simulink model "DA62_control"  (R2021a)
settings: Solver=ode4  StartTime=0.0  StopTime=300  FixedStep=0.001  RelTol=1e-3
InitFcn:
  | run('Stability_DA62')
values from neighbouring files (symbols this model uses):
  A = [Xu Xw 0 -g; Zu Zw U1 0; Mu+Mwdot*Zu Mw+Mwdot*Zw Mq+Mwdot*U1 0; 0 0 1 0]    [Stability_DA62.m]
  A_Lateral = [ Y_beta/U1 Y_p/U1 -(1-(Y_r/U1)) g*cosd(2)/U1 0; L_beta L_p L_r 0 0; N_beta N_p N_r 0 0; 0 1 0 0 0;0 0 1 0 0]    [Stability_DA62.m]
  B = [XdeltaE ;ZdeltaE; MdeltaE+Mwdot*ZdeltaE; 0]    [Stability_DA62.m]
  B_lateral = [Ydelta_a/U1 Ydelta_r/U1;Ldelta_a Ldelta_r; Ndelta_a Ndelta_r; 0 0;0 0 ]    [Stability_DA62.m]
  C_lateral = eye(5)    [Stability_DA62.m]
undefined symbols (not defined in the file or in its folder): Klqrgains
libraries: pid_lib x1
settings Model: Creator=IT-Defenders  LastModifiedBy=IT-Defenders

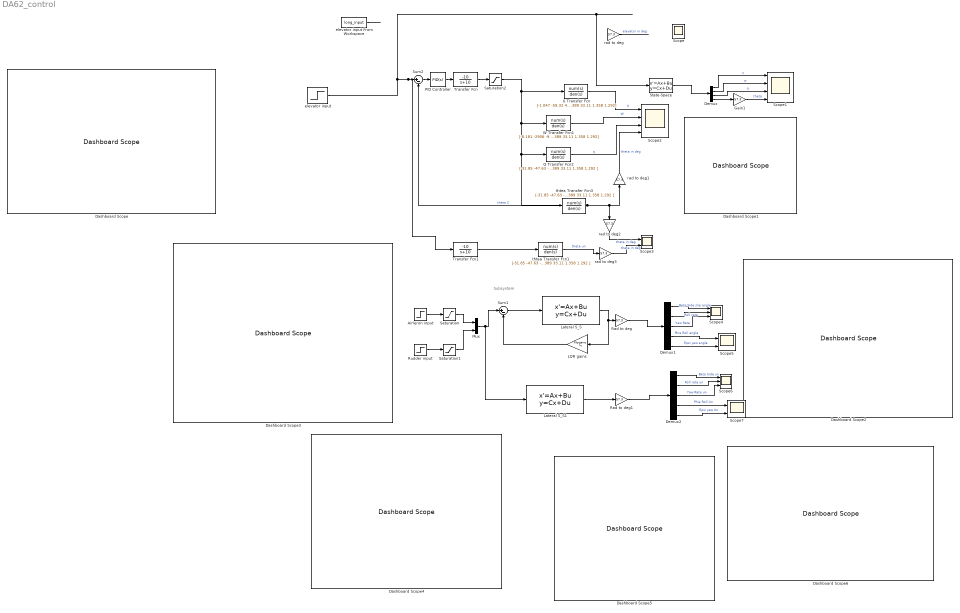
== system DA62_control ==
  note: Subsystem
  Airleron input : Step  After=20*pi/180  SampleTime=0
  Dashboard Scope{,1..6} (7 alike) : DashboardScope
  Demux : Demux
  Demux1 : Demux  Outputs=5
  Demux2 : Demux  Outputs=5
  Gain1 : Gain  Gain=57.3
  LQR gains : Gain  Gain=Klqrgains  Multiplication=Matrix(K*u)
  Lateral S_S : StateSpace  A=A_Lateral  B=B_lateral  C=C_lateral  D=zeros(5,2)  InitialCondition=0
  Lateral S_S1 : StateSpace  A=A_Lateral  B=B_lateral  C=C_lateral  D=zeros(5,2)  InitialCondition=0
  Mux : Mux  Inputs=2
  PID Controller : pid_lib/PID Controller  Controller=PID  Form=Parallel  TimeDomain=Continuous-time  UseExternalTs=off  SampleTime=-1  IntegratorMethod=Forward Euler  FilterMethod=Forward Euler  ControllerParametersSource=internal  P=0.880006891357761  I=0.782288298555866  D=-0.00238096460358231  UseFilter=on  N=369.600997021852  TunerSelectOption=Transfer Function Based (PID Tuner App)  InitialConditionSource=internal  InitialConditionForIntegrator=0  InitialConditionForFilter=0  DifferentiatorICPrevScaledInput=0  ExternalReset=none  TrackingMode=off  Kt=1  LimitOutput=off  SatLimitsSource=internal  UpperSaturationLimit=inf  LowerSaturationLimit=-inf  LinearizeAsGain=on  AntiWindupMode=none  Kb=1  POutMin=[]  POutMax=[]  IOutMin=[]  IOutMax=[]  DOutMin=[]  DOutMax=[]  NOutMin=[]  NOutMax=[]  SumOutMin=[]  SumOutMax=[]  SaturationOutMin=[]  SaturationOutMax=[]  PParamMin=[]  PParamMax=[]  IParamMin=[]  IParamMax=[]  DParamMin=[]  DParamMax=[]  NParamMin=[]  NParamMax=[]  KbParamMin=[]  KbParamMax=[]  KtParamMin=[]  KtParamMax=[]  KbOutMin=[]  KbOutMax=[]  KtOutMin=[]  KtOutMax=[]  IntegratorOutMin=[]  IntegratorOutMax=[]  FilterOutMin=[]  FilterOutMax=[]  SumI1OutMin=[]  SumI1OutMax=[]  SumI2OutMin=[]  SumI2OutMax=[]  SumI3OutMin=[]  SumI3OutMax=[]  SumI4OutMin=[]  SumI4OutMax=[]  SumDOutMin=[]  SumDOutMax=[]  DifferentiatorOutMin=[]  DifferentiatorOutMax=[]  FilterDiffOutCoefMin=[]  FilterDiffOutCoefMax=[]  ReciprocalOutMin=[]  ReciprocalOutMax=[]  SumDenOutMin=[]  SumDenOutMax=[]  SumNumOutMin=[]  SumNumOutMax=[]  DivideOutMin=[]  DivideOutMax=[]  UdiffTsProdOutMin=[]  UdiffTsProdOutMax=[]  NTsProdOutMin=[]  NTsProdOutMax=[]  UintegralTsProdOutMin=[]  UintegralTsProdOutMax=[]  UngainTsProdOutMin=[]  UngainTsProdOutMax=[]  IntegratorContinuousStateAttributes=''  IntegratorStateMustResolveToSignalObject=off  IntegratorRTWStateStorageClass=Auto  FilterContinuousStateAttributes=''  FilterStateMustResolveToSignalObject=off  FilterRTWStateStorageClass=Auto  ParallelPVariant=InternalParameters  IdealPVariant=Disabled  IVariant=InternalParameters  DVariant=InternalParameters  IntegratorVariant=Continuous  SatVariant=Disabled  AWVariant=Passthrough  PCopyVariant=Disabled  TRVariant=Disabled  FdbkBlocksVariant=Forward  IdealPFdbkVariant=Disabled  SatFdbkVariant=Disabled  DerivativeFilterVariant=ContFilter  NVariant=InternalParameters  NCopyVariant=Disabled  FilterICVariant=InternalICsFilter  IntegratorICVariant=InternalICs  ExternalResetVariant=Disabled  TRSumVariant=Passthrough  SumFdbkVariant=Disabled  SumVariant=Sum_PID  TsampFilterVariant=InternalTs  TsampNgainVariant=Passthrough  TsampIntegralVariant=Passthrough  ExternalSaturationOutDataTypeStr=Inherit: Same as second input
  Q Transfer Fcn2 : TransferFcn  Numerator=[-31.85 -47.63 -3.34 0]  Denominator=[1 6.389 33.11 1.358 1.292 ]
  Rad to deg : Gain  Gain=57.3
  Rad to deg1 : Gain  Gain=57.3
  Rudder input : Step  After=30*pi/180  SampleTime=0
  Saturation : Saturate  UpperLimit=50*pi/180  LowerLimit=-50*pi/180
  Saturation1 : Saturate  UpperLimit=30*pi/180  LowerLimit=-30*pi/180
  Saturation2 : Saturate  UpperLimit=15*pi/180  LowerLimit=-18*pi/180
  Scope{,3,5,7} (4 alike) : Scope  NumInputPorts=2
  Scope1 : Scope  NumInputPorts=4
  Scope2 : Scope  NumInputPorts=4
  Scope4 : Scope  NumInputPorts=3
  Scope6 : Scope  NumInputPorts=3
  State-Space : StateSpace  A=A  B=B  C=eye(4)  D=[0;0;0;0]  InitialCondition=0
  Sum1 : Sum  Inputs=|+-
  Sum2 : Sum  Inputs=|+-
  Transfer Fcn : TransferFcn  Numerator=[-10]  Denominator=[1 10]
  Transfer Fcn1 : TransferFcn  Numerator=[-10]  Denominator=[1 10]
  U Transfer Fcn : TransferFcn  Numerator=[-1.047 -59.32 456.8]  Denominator=[1 6.389 33.11 1.358 1.292]
  W Transfer Fcn1 : TransferFcn  Numerator=[-8.181 -2906 -97.1 -136.8 ]  Denominator=[1 6.389 33.11 1.358 1.292]
  elevator input : Step  After=-10*pi/180  SampleTime=0
  elevator input From Workspace : FromWorkspace  VariableName=long_input  SampleTime=1  OutputAfterFinalValue=Setting to zero
  rad to deg{,1..3} (4 alike) : Gain  Gain=57.3
  thtea Transfer Fcn1 : TransferFcn  Numerator=[-31.85 -47.63 -3.34]  Denominator=[1 6.389 33.11 1.358 1.292 ]
  thtea Transfer Fcn3 : TransferFcn  Numerator=[-31.85 -47.63 -3.34]  Denominator=[1 6.389 33.11 1.358 1.292 ]
  wires:
  State-Space/1 -> Demux/1
  Demux/4 -> Gain1/1
  Demux/1 -> Scope1/1  "u"
  Demux/2 -> Scope1/2  "w"
  Demux/3 -> Scope1/3  "q"
  Gain1/1 -> Scope1/4  "theta"
  rad to deg/1 -> ?  "elevator in deg"
  U Transfer Fcn/1 -> Scope2/1  "U"
  W Transfer Fcn1/1 -> Scope2/2  "W"
  thtea Transfer Fcn3/1 -> rad to deg1/1, rad to deg2/1, Sum2/2  "theta C"
  rad to deg1/1 -> Scope2/4  "theta in deg"
  Q Transfer Fcn2/1 -> Scope2/3  "q"
  Saturation2/1 -> thtea Transfer Fcn3/1, Q Transfer Fcn2/1, W Transfer Fcn1/1, U Transfer Fcn/1
  thtea Transfer Fcn1/1 -> rad to deg3/1  "theta un"
  Demux1/1 -> Scope4/1  "Beta Side slip angle"
  Demux1/2 -> Scope4/2  "Roll rate"
  Demux1/3 -> Scope4/3  "Yaw Rate"
  Demux1/4 -> Scope5/1  "Phie Roll angle"
  Airleron input/1 -> Saturation/1
  Rudder input/1 -> Saturation1/1
  Demux1/5 -> Scope5/2  "Epsi yaw angle"
  Saturation/1 -> Mux/1
  Saturation1/1 -> Mux/2
  Rad to deg/1 -> Demux1/1
  Mux/1 -> Lateral S_S1/1, Sum1/1
  LQR gains/1 -> Sum1/2
  Sum1/1 -> Lateral S_S/1
  Lateral S_S/1 -> LQR gains/1, Rad to deg/1
  Lateral S_S1/1 -> Rad to deg1/1
  Demux2/1 -> Scope6/1  "Beta Side un"
  Demux2/2 -> Scope6/2  "Roll rate un"
  Demux2/3 -> Scope6/3  "Yaw Rate un"
  Demux2/4 -> Scope7/1  "Phie Roll Un"
  Demux2/5 -> Scope7/2  "Epsi yaw Un"
  elevator input From Workspace/1 -> ?
  Rad to deg1/1 -> Demux2/1
  rad to deg2/1 -> Scope3/1  "theta in deg"
  rad to deg3/1 -> Scope3/2  "theta in deg"
  Transfer Fcn/1 -> Saturation2/1
  Sum2/1 -> PID Controller/1
  PID Controller/1 -> Transfer Fcn/1
  Transfer Fcn1/1 -> thtea Transfer Fcn1/1
  elevator input/1 -> State-Space/1, Transfer Fcn1/1, Sum2/1
